simulink model "ECU_B_Enumerated_Error_Code_Generator"  (R2022a)
settings: Solver=VariableStepAuto  StartTime=0.0  StopTime=10  RelTol=1e-3
(part 1 of 2)
settings Model: Creator=maxju  LastModifiedBy=maxju

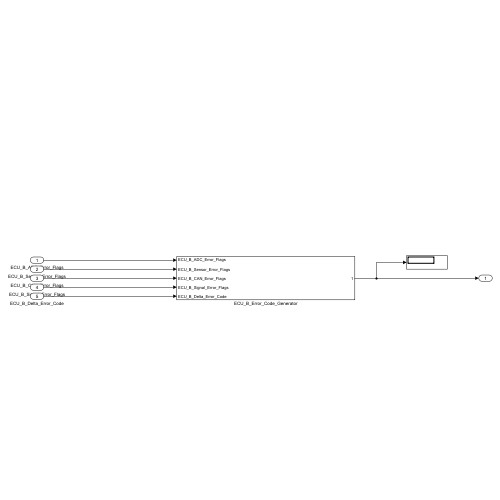
[thumbnail: Simulink's stored preview of the top-level diagram]
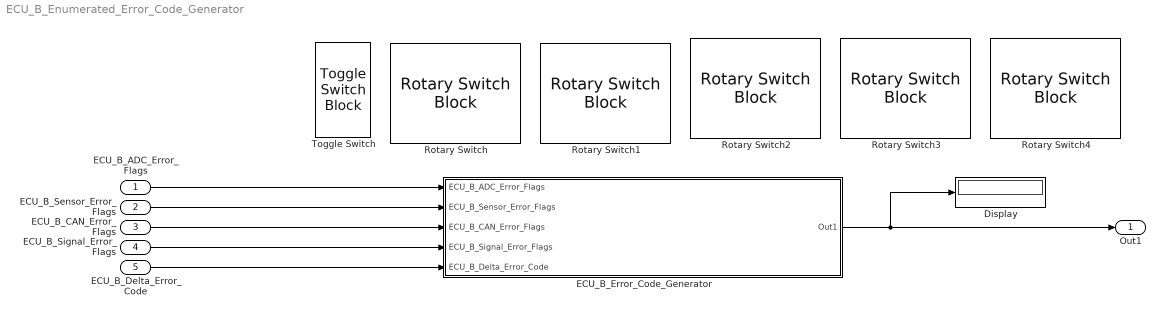
== system ECU_B_Enumerated_Error_Code_Generator ==
  ECU_B_ADC_Error_Flags : Inport
  ECU_B_Sensor_Error_Flags : Inport  Port=2
  ECU_B_CAN_Error_Flags : Inport  Port=3
  ECU_B_Signal_Error_Flags : Inport  Port=4
  ECU_B_Delta_Error_Code : Inport  Port=5
  Display : Display
  ECU_B_Error_Code_Generator : Subsystem
  Rotary Switch{,1..4} (5 alike) : RotarySwitchBlock
  Toggle Switch : ToggleSwitchBlock
      settings: Values={{'Off', 'On'}, [0 1]}
  Out1 : Outport
  wires:
  ECU_B_Signal_Error_Flags/1 -> ECU_B_Error_Code_Generator/4(ECU_B_Signal_Error_Flags)
  ECU_B_CAN_Error_Flags/1 -> ECU_B_Error_Code_Generator/3(ECU_B_CAN_Error_Flags)
  ECU_B_Sensor_Error_Flags/1 -> ECU_B_Error_Code_Generator/2(ECU_B_Sensor_Error_Flags)
  ECU_B_Error_Code_Generator/1(Out1) -> Out1/1, Display/1
  ECU_B_Delta_Error_Code/1 -> ECU_B_Error_Code_Generator/5(ECU_B_Delta_Error_Code)
  ECU_B_ADC_Error_Flags/1 -> ECU_B_Error_Code_Generator/1(ECU_B_ADC_Error_Flags)

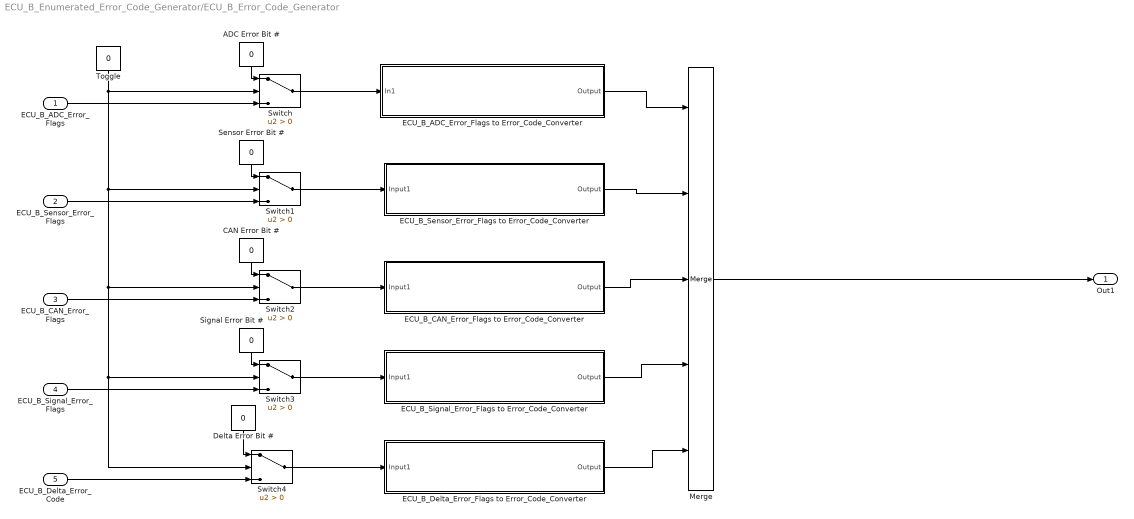
== system ECU_B_Enumerated_Error_Code_Generator/ECU_B_Error_Code_Generator ==
  ECU_B_ADC_Error_Flags : Inport
  ECU_B_Sensor_Error_Flags : Inport  Port=2
  ECU_B_CAN_Error_Flags : Inport  Port=3
  ECU_B_Signal_Error_Flags : Inport  Port=4
  ECU_B_Delta_Error_Code : Inport  Port=5
  ADC Error Bit # : Constant  Value=0
  CAN Error Bit # : Constant  Value=0
  Delta Error Bit # : Constant  Value=0
  ECU_B_ADC_Error_Flags to Error_Code_Converter : Subsystem
  ECU_B_CAN_Error_Flags to Error_Code_Converter : Subsystem
  ECU_B_Delta_Error_Flags to Error_Code_Converter : Subsystem
  ECU_B_Sensor_Error_Flags to Error_Code_Converter : Subsystem
  ECU_B_Signal_Error_Flags to Error_Code_Converter : Subsystem
  Merge : Merge  Inputs=5
  Sensor Error Bit # : Constant  Value=0
  Signal Error Bit # : Constant  Value=0
  Switch{,1..4} (5 alike) : Switch  Criteria=u2 > Threshold  SaturateOnIntegerOverflow=off  InputSameDT=off
  Toggle : Constant  Value=0
  Out1 : Outport
  wires:
  Merge/1 -> Out1/1
  ECU_B_ADC_Error_Flags to Error_Code_Converter/1(Output) -> Merge/1
  CAN Error Bit #/1 -> Switch2/1
  Switch1/1 -> ECU_B_Sensor_Error_Flags to Error_Code_Converter/1(Input1)
  Toggle/1 -> Switch2/2, Switch3/2, Switch4/2, Switch1/2, Switch/2
  ECU_B_Sensor_Error_Flags to Error_Code_Converter/1(Output) -> Merge/2
  ECU_B_CAN_Error_Flags to Error_Code_Converter/1(Output) -> Merge/3
  Switch/1 -> ECU_B_ADC_Error_Flags to Error_Code_Converter/1(In1)
  ECU_B_Signal_Error_Flags to Error_Code_Converter/1(Output) -> Merge/4
  Delta Error Bit #/1 -> Switch4/1
  ADC Error Bit #/1 -> Switch/1
  ECU_B_Delta_Error_Flags to Error_Code_Converter/1(Output) -> Merge/5
  ECU_B_Sensor_Error_Flags/1 -> Switch1/3
  ECU_B_ADC_Error_Flags/1 -> Switch/3
  Sensor Error Bit #/1 -> Switch1/1
  Signal Error Bit #/1 -> Switch3/1
  Switch2/1 -> ECU_B_CAN_Error_Flags to Error_Code_Converter/1(Input1)
  Switch3/1 -> ECU_B_Signal_Error_Flags to Error_Code_Converter/1(Input1)
  Switch4/1 -> ECU_B_Delta_Error_Flags to Error_Code_Converter/1(Input1)
  ECU_B_Signal_Error_Flags/1 -> Switch3/3
  ECU_B_CAN_Error_Flags/1 -> Switch2/3
  ECU_B_Delta_Error_Code/1 -> Switch4/3

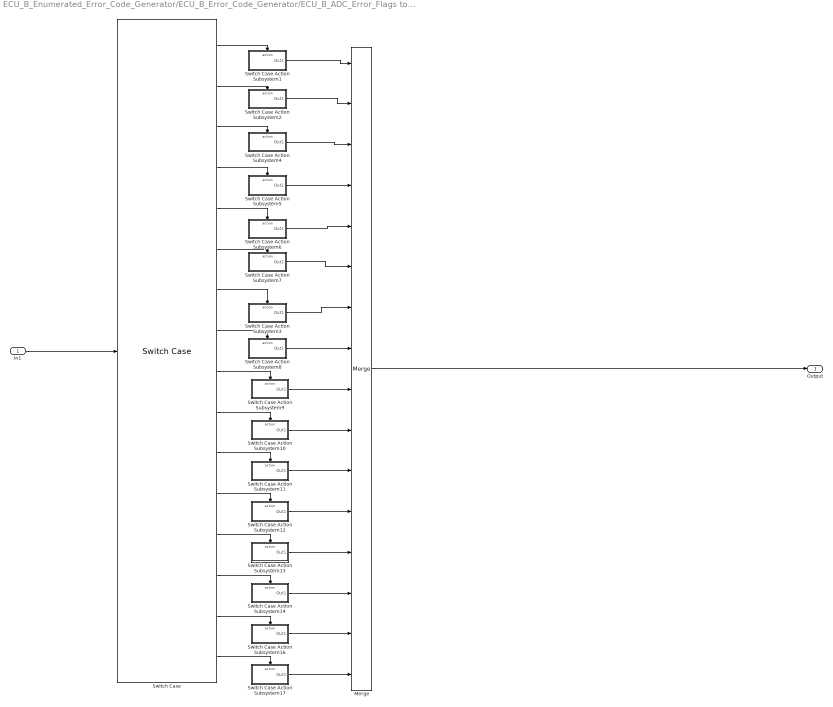
== system ECU_B_Enumerated_Error_Code_Generator/ECU_B_Error_Code_Generator/ECU_B_ADC_Error_Flags to Error_Code_Converter ==
  In1 : Inport
  Merge : Merge  Inputs=16
  Switch Case : SwitchCase  CaseConditions={1,2,3,4,5,6,7,8,9,10,11,12,13,14,15,16}  ShowDefaultCase=off
  Switch Case Action Subsystem1 : Subsystem  TreatAsAtomicUnit=on
  Switch Case Action Subsystem10 : Subsystem  TreatAsAtomicUnit=on
  Switch Case Action Subsystem11 : Subsystem  TreatAsAtomicUnit=on
  Switch Case Action Subsystem12 : Subsystem  TreatAsAtomicUnit=on
  Switch Case Action Subsystem13 : Subsystem  TreatAsAtomicUnit=on
  Switch Case Action Subsystem14 : Subsystem  TreatAsAtomicUnit=on
  Switch Case Action Subsystem16 : Subsystem  TreatAsAtomicUnit=on
  Switch Case Action Subsystem17 : Subsystem  TreatAsAtomicUnit=on
  Switch Case Action Subsystem2 : Subsystem  TreatAsAtomicUnit=on
  Switch Case Action Subsystem3 : Subsystem  TreatAsAtomicUnit=on
  Switch Case Action Subsystem4 : Subsystem  TreatAsAtomicUnit=on
  Switch Case Action Subsystem5 : Subsystem  TreatAsAtomicUnit=on
  Switch Case Action Subsystem6 : Subsystem  TreatAsAtomicUnit=on
  Switch Case Action Subsystem7 : Subsystem  TreatAsAtomicUnit=on
  Switch Case Action Subsystem8 : Subsystem  TreatAsAtomicUnit=on
  Switch Case Action Subsystem9 : Subsystem  TreatAsAtomicUnit=on
  Output : Outport
  wires:
  Switch Case/1 -> Switch Case Action Subsystem1/Action
  Switch Case/11 -> Switch Case Action Subsystem11/Action
  Switch Case/15 -> Switch Case Action Subsystem16/Action
  Switch Case Action Subsystem12/1(Out1) -> Merge/12
  Switch Case Action Subsystem17/1(Out1) -> Merge/16
  Switch Case/8 -> Switch Case Action Subsystem8/Action
  Switch Case Action Subsystem3/1(Out1) -> Merge/7
  Switch Case Action Subsystem14/1(Out1) -> Merge/14
  Switch Case/2 -> Switch Case Action Subsystem2/Action
  Switch Case/6 -> Switch Case Action Subsystem7/Action
  Switch Case Action Subsystem8/1(Out1) -> Merge/8
  Switch Case Action Subsystem10/1(Out1) -> Merge/10
  Switch Case Action Subsystem1/1(Out1) -> Merge/1
  Switch Case/9 -> Switch Case Action Subsystem9/Action
  Switch Case Action Subsystem5/1(Out1) -> Merge/4
  Switch Case Action Subsystem13/1(Out1) -> Merge/13
  Switch Case Action Subsystem11/1(Out1) -> Merge/11
  Switch Case/16 -> Switch Case Action Subsystem17/Action
  In1/1 -> Switch Case/1
  Switch Case/3 -> Switch Case Action Subsystem4/Action
  Switch Case/4 -> Switch Case Action Subsystem5/Action
  Switch Case/14 -> Switch Case Action Subsystem14/Action
  Switch Case Action Subsystem6/1(Out1) -> Merge/5
  Switch Case/5 -> Switch Case Action Subsystem6/Action
  Switch Case Action Subsystem2/1(Out1) -> Merge/2
  Switch Case/12 -> Switch Case Action Subsystem12/Action
  Switch Case Action Subsystem4/1(Out1) -> Merge/3
  Switch Case Action Subsystem9/1(Out1) -> Merge/9
  Switch Case/7 -> Switch Case Action Subsystem3/Action
  Switch Case/13 -> Switch Case Action Subsystem13/Action
  Switch Case Action Subsystem7/1(Out1) -> Merge/6
  Switch Case/10 -> Switch Case Action Subsystem10/Action
  Switch Case Action Subsystem16/1(Out1) -> Merge/15
  Merge/1 -> Output/1

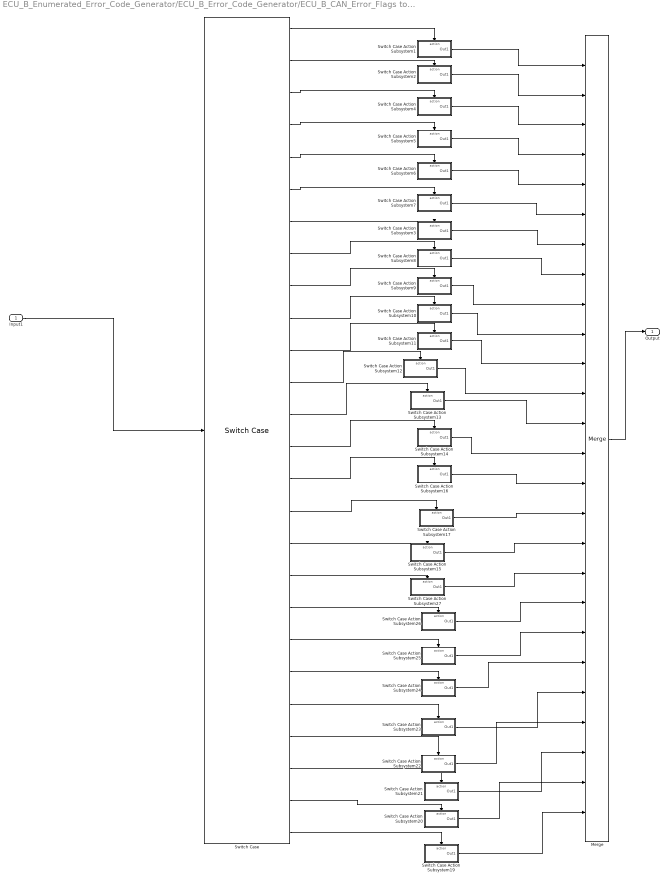
== system ECU_B_Enumerated_Error_Code_Generator/ECU_B_Error_Code_Generator/ECU_B_CAN_Error_Flags to Error_Code_Converter ==
  Input1 : Inport
  Merge : Merge  Inputs=26
  Switch Case : SwitchCase  CaseConditions={1,2,3,4,5,6,7,8,9,10,11,12,13,14,15,16,17,18,19,20,21,22,23,24,25,26}  ShowDefaultCase=off
  Switch Case Action Subsystem1 : Subsystem  TreatAsAtomicUnit=on
  Switch Case Action Subsystem10 : Subsystem  TreatAsAtomicUnit=on
  Switch Case Action Subsystem11 : Subsystem  TreatAsAtomicUnit=on
  Switch Case Action Subsystem12 : Subsystem  TreatAsAtomicUnit=on
  Switch Case Action Subsystem13 : Subsystem  TreatAsAtomicUnit=on
  Switch Case Action Subsystem14 : Subsystem  TreatAsAtomicUnit=on
  Switch Case Action Subsystem15 : Subsystem  TreatAsAtomicUnit=on
  Switch Case Action Subsystem16 : Subsystem  TreatAsAtomicUnit=on
  Switch Case Action Subsystem17 : Subsystem  TreatAsAtomicUnit=on
  Switch Case Action Subsystem19 : Subsystem  TreatAsAtomicUnit=on
  Switch Case Action Subsystem2 : Subsystem  TreatAsAtomicUnit=on
  Switch Case Action Subsystem20 : Subsystem  TreatAsAtomicUnit=on
  Switch Case Action Subsystem21 : Subsystem  TreatAsAtomicUnit=on
  Switch Case Action Subsystem22 : Subsystem  TreatAsAtomicUnit=on
  Switch Case Action Subsystem23 : Subsystem  TreatAsAtomicUnit=on
  Switch Case Action Subsystem24 : Subsystem  TreatAsAtomicUnit=on
  Switch Case Action Subsystem25 : Subsystem  TreatAsAtomicUnit=on
  Switch Case Action Subsystem26 : Subsystem  TreatAsAtomicUnit=on
  Switch Case Action Subsystem27 : Subsystem  TreatAsAtomicUnit=on
  Switch Case Action Subsystem3 : Subsystem  TreatAsAtomicUnit=on
  Switch Case Action Subsystem4 : Subsystem  TreatAsAtomicUnit=on
  Switch Case Action Subsystem5 : Subsystem  TreatAsAtomicUnit=on
  Switch Case Action Subsystem6 : Subsystem  TreatAsAtomicUnit=on
  Switch Case Action Subsystem7 : Subsystem  TreatAsAtomicUnit=on
  Switch Case Action Subsystem8 : Subsystem  TreatAsAtomicUnit=on
  Switch Case Action Subsystem9 : Subsystem  TreatAsAtomicUnit=on
  Output : Outport
  wires:
  Switch Case/1 -> Switch Case Action Subsystem1/Action
  Switch Case/11 -> Switch Case Action Subsystem11/Action
  Switch Case/15 -> Switch Case Action Subsystem16/Action
  Switch Case Action Subsystem12/1(Out1) -> Merge/12
  Switch Case Action Subsystem17/1(Out1) -> Merge/16
  Switch Case/8 -> Switch Case Action Subsystem8/Action
  Switch Case Action Subsystem3/1(Out1) -> Merge/7
  Switch Case Action Subsystem14/1(Out1) -> Merge/14
  Switch Case/2 -> Switch Case Action Subsystem2/Action
  Switch Case/6 -> Switch Case Action Subsystem7/Action
  Switch Case Action Subsystem8/1(Out1) -> Merge/8
  Switch Case Action Subsystem10/1(Out1) -> Merge/10
  Switch Case Action Subsystem1/1(Out1) -> Merge/1
  Switch Case/9 -> Switch Case Action Subsystem9/Action
  Switch Case Action Subsystem5/1(Out1) -> Merge/4
  Switch Case Action Subsystem13/1(Out1) -> Merge/13
  Switch Case Action Subsystem11/1(Out1) -> Merge/11
  Merge/1 -> Output/1
  Switch Case/16 -> Switch Case Action Subsystem17/Action
  Input1/1 -> Switch Case/1
  Switch Case/3 -> Switch Case Action Subsystem4/Action
  Switch Case/4 -> Switch Case Action Subsystem5/Action
  Switch Case/14 -> Switch Case Action Subsystem14/Action
  Switch Case Action Subsystem6/1(Out1) -> Merge/5
  Switch Case/5 -> Switch Case Action Subsystem6/Action
  Switch Case Action Subsystem2/1(Out1) -> Merge/2
  Switch Case/12 -> Switch Case Action Subsystem12/Action
  Switch Case Action Subsystem4/1(Out1) -> Merge/3
  Switch Case Action Subsystem9/1(Out1) -> Merge/9
  Switch Case/7 -> Switch Case Action Subsystem3/Action
  Switch Case/13 -> Switch Case Action Subsystem13/Action
  Switch Case Action Subsystem7/1(Out1) -> Merge/6
  Switch Case/10 -> Switch Case Action Subsystem10/Action
  Switch Case Action Subsystem16/1(Out1) -> Merge/15
  Switch Case/17 -> Switch Case Action Subsystem15/Action
  Switch Case Action Subsystem15/1(Out1) -> Merge/17
  Switch Case/18 -> Switch Case Action Subsystem27/Action
  Switch Case Action Subsystem27/1(Out1) -> Merge/18
  Switch Case/19 -> Switch Case Action Subsystem26/Action
  Switch Case Action Subsystem26/1(Out1) -> Merge/19
  Switch Case/20 -> Switch Case Action Subsystem25/Action
  Switch Case Action Subsystem25/1(Out1) -> Merge/20
  Switch Case/21 -> Switch Case Action Subsystem24/Action
  Switch Case Action Subsystem24/1(Out1) -> Merge/21
  Switch Case/22 -> Switch Case Action Subsystem23/Action
  Switch Case Action Subsystem23/1(Out1) -> Merge/22
  Switch Case/23 -> Switch Case Action Subsystem22/Action
  Switch Case Action Subsystem22/1(Out1) -> Merge/23
  Switch Case/24 -> Switch Case Action Subsystem21/Action
  Switch Case Action Subsystem21/1(Out1) -> Merge/24
  Switch Case/25 -> Switch Case Action Subsystem20/Action
  Switch Case Action Subsystem20/1(Out1) -> Merge/25
  Switch Case/26 -> Switch Case Action Subsystem19/Action
  Switch Case Action Subsystem19/1(Out1) -> Merge/26

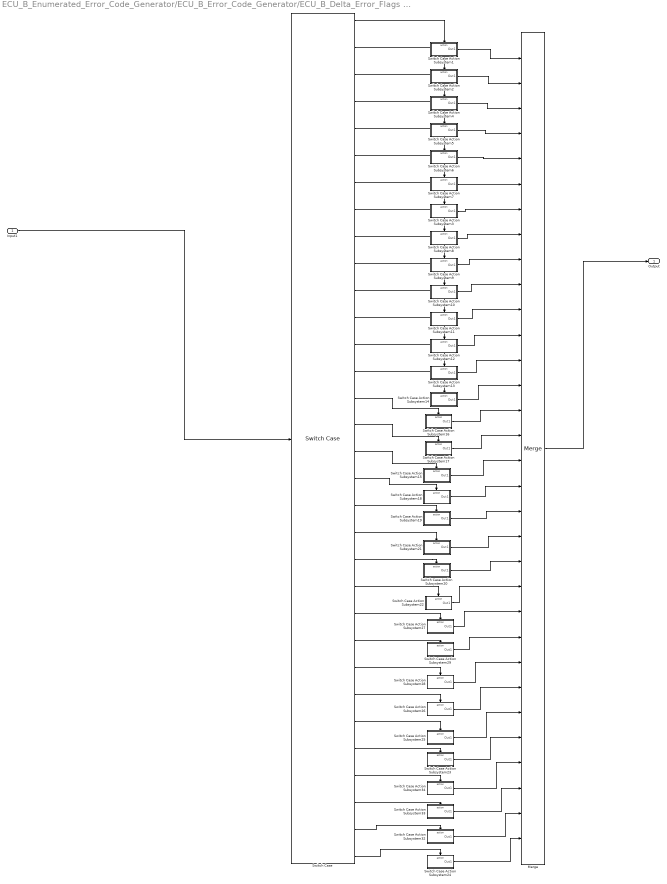
== system ECU_B_Enumerated_Error_Code_Generator/ECU_B_Error_Code_Generator/ECU_B_Delta_Error_Flags to Error_Code_Converter ==
  Input1 : Inport
  Merge : Merge  Inputs=32
  Switch Case : SwitchCase  CaseConditions={1,2,3,4,5,6,7,8,9,10,11,12,13,14,15,16,17,18,19,20,21,22,23,24,25,26,27,28,29,30,31,32}  ShowDefaultCase=off
  Switch Case Action Subsystem1 : Subsystem  TreatAsAtomicUnit=on
  Switch Case Action Subsystem10 : Subsystem  TreatAsAtomicUnit=on
  Switch Case Action Subsystem11 : Subsystem  TreatAsAtomicUnit=on
  Switch Case Action Subsystem12 : Subsystem  TreatAsAtomicUnit=on
  Switch Case Action Subsystem13 : Subsystem  TreatAsAtomicUnit=on
  Switch Case Action Subsystem14 : Subsystem  TreatAsAtomicUnit=on
  Switch Case Action Subsystem15 : Subsystem  TreatAsAtomicUnit=on
  Switch Case Action Subsystem16 : Subsystem  TreatAsAtomicUnit=on
  Switch Case Action Subsystem17 : Subsystem  TreatAsAtomicUnit=on
  Switch Case Action Subsystem18 : Subsystem  TreatAsAtomicUnit=on
  Switch Case Action Subsystem19 : Subsystem  TreatAsAtomicUnit=on
  Switch Case Action Subsystem2 : Subsystem  TreatAsAtomicUnit=on
  Switch Case Action Subsystem20 : Subsystem  TreatAsAtomicUnit=on
  Switch Case Action Subsystem21 : Subsystem  TreatAsAtomicUnit=on
  Switch Case Action Subsystem22 : Subsystem  TreatAsAtomicUnit=on
  Switch Case Action Subsystem23 : Subsystem  TreatAsAtomicUnit=on
  Switch Case Action Subsystem24 : Subsystem  TreatAsAtomicUnit=on
  Switch Case Action Subsystem25 : Subsystem  TreatAsAtomicUnit=on
  Switch Case Action Subsystem26 : Subsystem  TreatAsAtomicUnit=on
  Switch Case Action Subsystem27 : Subsystem  TreatAsAtomicUnit=on
  Switch Case Action Subsystem28 : Subsystem  TreatAsAtomicUnit=on
  Switch Case Action Subsystem29 : Subsystem  TreatAsAtomicUnit=on
  Switch Case Action Subsystem3 : Subsystem  TreatAsAtomicUnit=on
  Switch Case Action Subsystem32 : Subsystem  TreatAsAtomicUnit=on
  Switch Case Action Subsystem33 : Subsystem  TreatAsAtomicUnit=on
  Switch Case Action Subsystem34 : Subsystem  TreatAsAtomicUnit=on
  Switch Case Action Subsystem4 : Subsystem  TreatAsAtomicUnit=on
  Switch Case Action Subsystem5 : Subsystem  TreatAsAtomicUnit=on
  Switch Case Action Subsystem6 : Subsystem  TreatAsAtomicUnit=on
  Switch Case Action Subsystem7 : Subsystem  TreatAsAtomicUnit=on
  Switch Case Action Subsystem8 : Subsystem  TreatAsAtomicUnit=on
  Switch Case Action Subsystem9 : Subsystem  TreatAsAtomicUnit=on
  Output : Outport
  wires:
  Switch Case/1 -> Switch Case Action Subsystem1/Action
  Switch Case/11 -> Switch Case Action Subsystem11/Action
  Switch Case/15 -> Switch Case Action Subsystem16/Action
  Switch Case Action Subsystem12/1(Out1) -> Merge/12
  Switch Case Action Subsystem17/1(Out1) -> Merge/16
  Switch Case/8 -> Switch Case Action Subsystem8/Action
  Switch Case Action Subsystem3/1(Out1) -> Merge/7
  Switch Case Action Subsystem14/1(Out1) -> Merge/14
  Switch Case/2 -> Switch Case Action Subsystem2/Action
  Switch Case/6 -> Switch Case Action Subsystem7/Action
  Switch Case Action Subsystem8/1(Out1) -> Merge/8
  Switch Case Action Subsystem10/1(Out1) -> Merge/10
  Switch Case Action Subsystem1/1(Out1) -> Merge/1
  Switch Case/9 -> Switch Case Action Subsystem9/Action
  Switch Case Action Subsystem5/1(Out1) -> Merge/4
  Switch Case Action Subsystem13/1(Out1) -> Merge/13
  Switch Case Action Subsystem11/1(Out1) -> Merge/11
  Merge/1 -> Output/1
  Switch Case/16 -> Switch Case Action Subsystem17/Action
  Input1/1 -> Switch Case/1
  Switch Case/3 -> Switch Case Action Subsystem4/Action
  Switch Case/4 -> Switch Case Action Subsystem5/Action
  Switch Case/14 -> Switch Case Action Subsystem14/Action
  Switch Case Action Subsystem6/1(Out1) -> Merge/5
  Switch Case/5 -> Switch Case Action Subsystem6/Action
  Switch Case Action Subsystem2/1(Out1) -> Merge/2
  Switch Case/12 -> Switch Case Action Subsystem12/Action
  Switch Case Action Subsystem4/1(Out1) -> Merge/3
  Switch Case Action Subsystem9/1(Out1) -> Merge/9
  Switch Case/7 -> Switch Case Action Subsystem3/Action
  Switch Case/13 -> Switch Case Action Subsystem13/Action
  Switch Case Action Subsystem7/1(Out1) -> Merge/6
  Switch Case/10 -> Switch Case Action Subsystem10/Action
  Switch Case Action Subsystem16/1(Out1) -> Merge/15
  Switch Case/17 -> Switch Case Action Subsystem15/Action
  Switch Case Action Subsystem15/1(Out1) -> Merge/17
  Switch Case/18 -> Switch Case Action Subsystem18/Action
  Switch Case Action Subsystem18/1(Out1) -> Merge/18
  Switch Case/19 -> Switch Case Action Subsystem19/Action
  Switch Case Action Subsystem19/1(Out1) -> Merge/19
  Switch Case/20 -> Switch Case Action Subsystem21/Action
  Switch Case Action Subsystem21/1(Out1) -> Merge/20
  Switch Case/21 -> Switch Case Action Subsystem20/Action
  Switch Case Action Subsystem20/1(Out1) -> Merge/21
  Switch Case/22 -> Switch Case Action Subsystem22/Action
  Switch Case Action Subsystem22/1(Out1) -> Merge/22
  Switch Case/23 -> Switch Case Action Subsystem27/Action
  Switch Case Action Subsystem27/1(Out1) -> Merge/23
  Switch Case/24 -> Switch Case Action Subsystem29/Action
  Switch Case Action Subsystem29/1(Out1) -> Merge/24
  Switch Case/25 -> Switch Case Action Subsystem28/Action
  Switch Case Action Subsystem28/1(Out1) -> Merge/25
  Switch Case/26 -> Switch Case Action Subsystem26/Action
  Switch Case Action Subsystem26/1(Out1) -> Merge/26
  Switch Case/27 -> Switch Case Action Subsystem25/Action
  Switch Case Action Subsystem25/1(Out1) -> Merge/27
  Switch Case/28 -> Switch Case Action Subsystem23/Action
  Switch Case Action Subsystem23/1(Out1) -> Merge/28
  Switch Case/29 -> Switch Case Action Subsystem34/Action
  Switch Case Action Subsystem34/1(Out1) -> Merge/29
  Switch Case/30 -> Switch Case Action Subsystem33/Action
  Switch Case Action Subsystem33/1(Out1) -> Merge/30
  Switch Case/31 -> Switch Case Action Subsystem32/Action
  Switch Case Action Subsystem32/1(Out1) -> Merge/31
  Switch Case/32 -> Switch Case Action Subsystem24/Action
  Switch Case Action Subsystem24/1(Out1) -> Merge/32

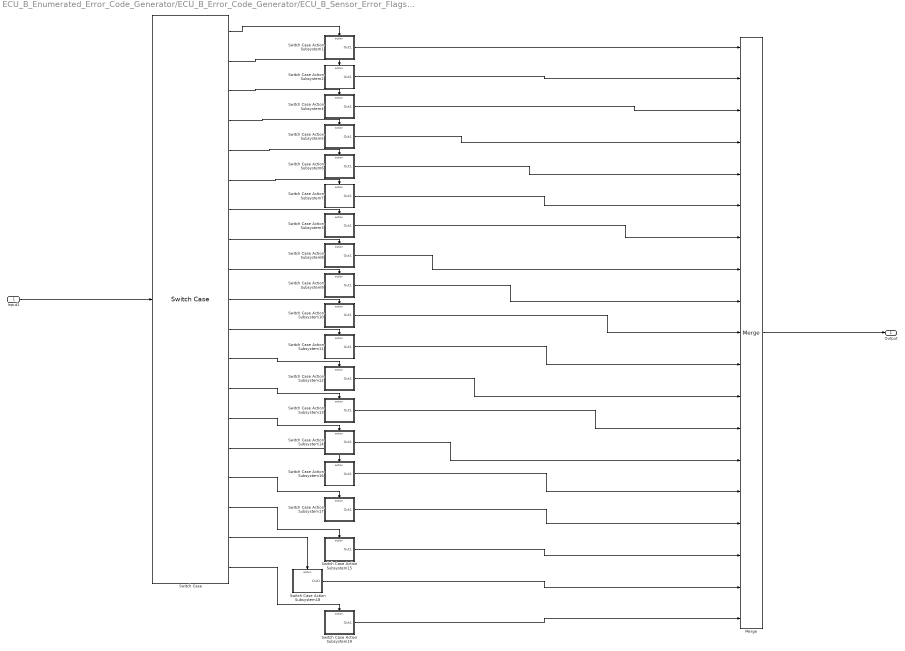
== system ECU_B_Enumerated_Error_Code_Generator/ECU_B_Error_Code_Generator/ECU_B_Sensor_Error_Flags to Error_Code_Converter ==
  Input1 : Inport
  Merge : Merge  Inputs=19
  Switch Case : SwitchCase  CaseConditions={1,2,3,4,5,6,7,8,9,10,11,12,13,14,15,16,17,18,19}  ShowDefaultCase=off
  Switch Case Action Subsystem1 : Subsystem  TreatAsAtomicUnit=on
  Switch Case Action Subsystem10 : Subsystem  TreatAsAtomicUnit=on
  Switch Case Action Subsystem11 : Subsystem  TreatAsAtomicUnit=on
  Switch Case Action Subsystem12 : Subsystem  TreatAsAtomicUnit=on
  Switch Case Action Subsystem13 : Subsystem  TreatAsAtomicUnit=on
  Switch Case Action Subsystem14 : Subsystem  TreatAsAtomicUnit=on
  Switch Case Action Subsystem15 : Subsystem  TreatAsAtomicUnit=on
  Switch Case Action Subsystem16 : Subsystem  TreatAsAtomicUnit=on
  Switch Case Action Subsystem17 : Subsystem  TreatAsAtomicUnit=on
  Switch Case Action Subsystem18 : Subsystem  TreatAsAtomicUnit=on
  Switch Case Action Subsystem19 : Subsystem  TreatAsAtomicUnit=on
  Switch Case Action Subsystem2 : Subsystem  TreatAsAtomicUnit=on
  Switch Case Action Subsystem3 : Subsystem  TreatAsAtomicUnit=on
  Switch Case Action Subsystem4 : Subsystem  TreatAsAtomicUnit=on
  Switch Case Action Subsystem5 : Subsystem  TreatAsAtomicUnit=on
  Switch Case Action Subsystem6 : Subsystem  TreatAsAtomicUnit=on
  Switch Case Action Subsystem7 : Subsystem  TreatAsAtomicUnit=on
  Switch Case Action Subsystem8 : Subsystem  TreatAsAtomicUnit=on
  Switch Case Action Subsystem9 : Subsystem  TreatAsAtomicUnit=on
  Output : Outport
  wires:
  Switch Case Action Subsystem5/1(Out1) -> Merge/4
  Switch Case Action Subsystem1/1(Out1) -> Merge/1
  Switch Case Action Subsystem17/1(Out1) -> Merge/16
  Switch Case Action Subsystem3/1(Out1) -> Merge/7
  Switch Case Action Subsystem10/1(Out1) -> Merge/10
  Switch Case Action Subsystem14/1(Out1) -> Merge/14
  Switch Case/2 -> Switch Case Action Subsystem2/Action
  Switch Case/1 -> Switch Case Action Subsystem1/Action
  Switch Case Action Subsystem13/1(Out1) -> Merge/13
  Switch Case Action Subsystem11/1(Out1) -> Merge/11
  Merge/1 -> Output/1
  Switch Case/15 -> Switch Case Action Subsystem16/Action
  Switch Case/16 -> Switch Case Action Subsystem17/Action
  Input1/1 -> Switch Case/1
  Switch Case/3 -> Switch Case Action Subsystem4/Action
  Switch Case/4 -> Switch Case Action Subsystem5/Action
  Switch Case Action Subsystem6/1(Out1) -> Merge/5
  Switch Case/6 -> Switch Case Action Subsystem7/Action
  Switch Case/5 -> Switch Case Action Subsystem6/Action
  Switch Case Action Subsystem2/1(Out1) -> Merge/2
  Switch Case/11 -> Switch Case Action Subsystem11/Action
  Switch Case/12 -> Switch Case Action Subsystem12/Action
  Switch Case Action Subsystem4/1(Out1) -> Merge/3
  Switch Case Action Subsystem9/1(Out1) -> Merge/9
  Switch Case/8 -> Switch Case Action Subsystem8/Action
  Switch Case/7 -> Switch Case Action Subsystem3/Action
  Switch Case/14 -> Switch Case Action Subsystem14/Action
  Switch Case/13 -> Switch Case Action Subsystem13/Action
  Switch Case Action Subsystem7/1(Out1) -> Merge/6
  Switch Case/17 -> Switch Case Action Subsystem15/Action
  Switch Case/19 -> Switch Case Action Subsystem19/Action
  Switch Case Action Subsystem18/1(Out1) -> Merge/18
  Switch Case Action Subsystem15/1(Out1) -> Merge/17
  Switch Case/9 -> Switch Case Action Subsystem9/Action
  Switch Case/10 -> Switch Case Action Subsystem10/Action
  Switch Case Action Subsystem12/1(Out1) -> Merge/12
  Switch Case Action Subsystem19/1(Out1) -> Merge/19
  Switch Case Action Subsystem8/1(Out1) -> Merge/8
  Switch Case/18 -> Switch Case Action Subsystem18/Action
  Switch Case Action Subsystem16/1(Out1) -> Merge/15

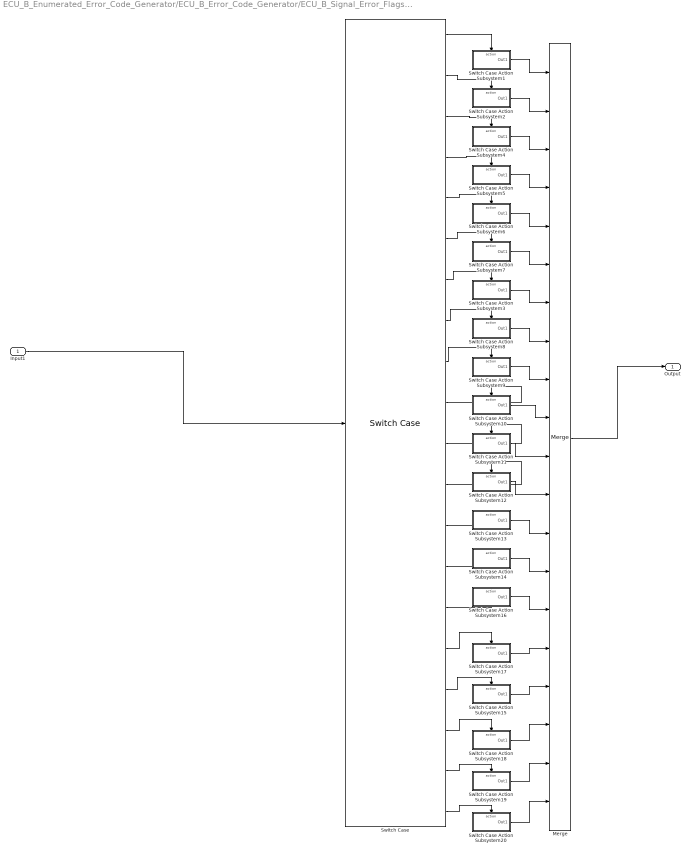
== system ECU_B_Enumerated_Error_Code_Generator/ECU_B_Error_Code_Generator/ECU_B_Signal_Error_Flags to Error_Code_Converter ==
  Input1 : Inport
  Merge : Merge  Inputs=20
  Switch Case : SwitchCase  CaseConditions={1,2,3,4,5,6,7,8,9,10,11,12,13,14,15,16,17,18,19,20}  ShowDefaultCase=off
  Switch Case Action Subsystem1 : Subsystem  TreatAsAtomicUnit=on
  Switch Case Action Subsystem10 : Subsystem  TreatAsAtomicUnit=on
  Switch Case Action Subsystem11 : Subsystem  TreatAsAtomicUnit=on
  Switch Case Action Subsystem12 : Subsystem  TreatAsAtomicUnit=on
  Switch Case Action Subsystem13 : Subsystem  TreatAsAtomicUnit=on
  Switch Case Action Subsystem14 : Subsystem  TreatAsAtomicUnit=on
  Switch Case Action Subsystem15 : Subsystem  TreatAsAtomicUnit=on
  Switch Case Action Subsystem16 : Subsystem  TreatAsAtomicUnit=on
  Switch Case Action Subsystem17 : Subsystem  TreatAsAtomicUnit=on
  Switch Case Action Subsystem18 : Subsystem  TreatAsAtomicUnit=on
  Switch Case Action Subsystem19 : Subsystem  TreatAsAtomicUnit=on
  Switch Case Action Subsystem2 : Subsystem  TreatAsAtomicUnit=on
  Switch Case Action Subsystem20 : Subsystem  TreatAsAtomicUnit=on
  Switch Case Action Subsystem3 : Subsystem  TreatAsAtomicUnit=on
  Switch Case Action Subsystem4 : Subsystem  TreatAsAtomicUnit=on
  Switch Case Action Subsystem5 : Subsystem  TreatAsAtomicUnit=on
  Switch Case Action Subsystem6 : Subsystem  TreatAsAtomicUnit=on
  Switch Case Action Subsystem7 : Subsystem  TreatAsAtomicUnit=on
  Switch Case Action Subsystem8 : Subsystem  TreatAsAtomicUnit=on
  Switch Case Action Subsystem9 : Subsystem  TreatAsAtomicUnit=on
  Output : Outport
  wires:
  Switch Case/1 -> Switch Case Action Subsystem1/Action
  Switch Case/11 -> Switch Case Action Subsystem11/Action
  Switch Case/15 -> Switch Case Action Subsystem16/Action
  Switch Case Action Subsystem12/1(Out1) -> Merge/12
  Switch Case Action Subsystem17/1(Out1) -> Merge/16
  Switch Case/8 -> Switch Case Action Subsystem8/Action
  Switch Case Action Subsystem3/1(Out1) -> Merge/7
  Switch Case Action Subsystem14/1(Out1) -> Merge/14
  Switch Case/2 -> Switch Case Action Subsystem2/Action
  Switch Case/6 -> Switch Case Action Subsystem7/Action
  Switch Case Action Subsystem8/1(Out1) -> Merge/8
  Switch Case Action Subsystem10/1(Out1) -> Merge/10
  Switch Case Action Subsystem1/1(Out1) -> Merge/1
  Switch Case/9 -> Switch Case Action Subsystem9/Action
  Switch Case Action Subsystem5/1(Out1) -> Merge/4
  Switch Case Action Subsystem13/1(Out1) -> Merge/13
  Switch Case Action Subsystem11/1(Out1) -> Merge/11
  Merge/1 -> Output/1
  Switch Case/16 -> Switch Case Action Subsystem17/Action
  Input1/1 -> Switch Case/1
  Switch Case/3 -> Switch Case Action Subsystem4/Action
  Switch Case/4 -> Switch Case Action Subsystem5/Action
  Switch Case/14 -> Switch Case Action Subsystem14/Action
  Switch Case Action Subsystem6/1(Out1) -> Merge/5
  Switch Case/5 -> Switch Case Action Subsystem6/Action
  Switch Case Action Subsystem2/1(Out1) -> Merge/2
  Switch Case/12 -> Switch Case Action Subsystem12/Action
  Switch Case Action Subsystem4/1(Out1) -> Merge/3
  Switch Case Action Subsystem9/1(Out1) -> Merge/9
  Switch Case/7 -> Switch Case Action Subsystem3/Action
  Switch Case/13 -> Switch Case Action Subsystem13/Action
  Switch Case Action Subsystem7/1(Out1) -> Merge/6
  Switch Case/10 -> Switch Case Action Subsystem10/Action
  Switch Case Action Subsystem16/1(Out1) -> Merge/15
  Switch Case/17 -> Switch Case Action Subsystem15/Action
  Switch Case/18 -> Switch Case Action Subsystem18/Action
  Switch Case/19 -> Switch Case Action Subsystem19/Action
  Switch Case/20 -> Switch Case Action Subsystem20/Action
  Switch Case Action Subsystem15/1(Out1) -> Merge/17
  Switch Case Action Subsystem18/1(Out1) -> Merge/18
  Switch Case Action Subsystem19/1(Out1) -> Merge/19
  Switch Case Action Subsystem20/1(Out1) -> Merge/20

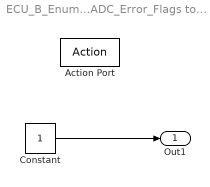
== system ECU_B_Enumerated_Error_Code_Generator/ECU_B_Error_Code_Generator/ECU_B_ADC_Error_Flags to Error_Code_Converter/Switch Case Action Subsystem1 ==
  Action Port : ActionPort  ActionPortLabel=case [ 1 ]:
  Constant : Constant
  Out1 : Outport  VectorParamsAs1DForOutWhenUnconnected=off
  wires:
  Constant/1 -> Out1/1

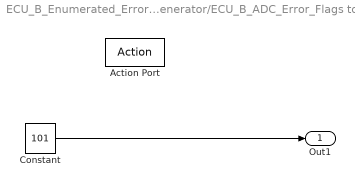
== system ECU_B_Enumerated_Error_Code_Generator/ECU_B_Error_Code_Generator/ECU_B_ADC_Error_Flags to Error_Code_Converter/Switch Case Action Subsystem10 ==
  Action Port : ActionPort  ActionPortLabel=case [ 10 ]:
  Constant : Constant  Value=101
  Out1 : Outport  VectorParamsAs1DForOutWhenUnconnected=off
  wires:
  Constant/1 -> Out1/1

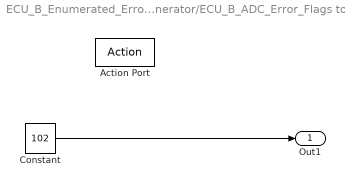
== system ECU_B_Enumerated_Error_Code_Generator/ECU_B_Error_Code_Generator/ECU_B_ADC_Error_Flags to Error_Code_Converter/Switch Case Action Subsystem11 ==
  Action Port : ActionPort  ActionPortLabel=case [ 11 ]:
  Constant : Constant  Value=102
  Out1 : Outport  VectorParamsAs1DForOutWhenUnconnected=off
  wires:
  Constant/1 -> Out1/1

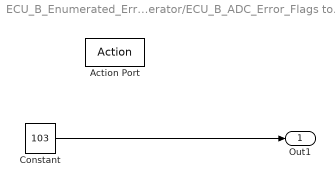
== system ECU_B_Enumerated_Error_Code_Generator/ECU_B_Error_Code_Generator/ECU_B_ADC_Error_Flags to Error_Code_Converter/Switch Case Action Subsystem12 ==
  Action Port : ActionPort  ActionPortLabel=case [ 12 ]:
  Constant : Constant  Value=103
  Out1 : Outport  VectorParamsAs1DForOutWhenUnconnected=off
  wires:
  Constant/1 -> Out1/1

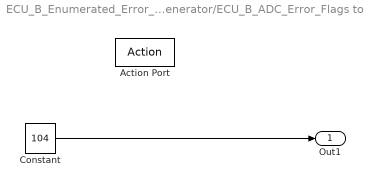
== system ECU_B_Enumerated_Error_Code_Generator/ECU_B_Error_Code_Generator/ECU_B_ADC_Error_Flags to Error_Code_Converter/Switch Case Action Subsystem13 ==
  Action Port : ActionPort  ActionPortLabel=case [ 13 ]:
  Constant : Constant  Value=104
  Out1 : Outport  VectorParamsAs1DForOutWhenUnconnected=off
  wires:
  Constant/1 -> Out1/1

== system ECU_B_Enumerated_Error_Code_Generator/ECU_B_Error_Code_Generator/ECU_B_ADC_Error_Flags to Error_Code_Converter/Switch Case Action Subsystem14 ==
  Action Port : ActionPort  ActionPortLabel=case [ 14 ]:
  Constant : Constant  Value=105
  Out1 : Outport  VectorParamsAs1DForOutWhenUnconnected=off
  wires:
  Constant/1 -> Out1/1

== system ECU_B_Enumerated_Error_Code_Generator/ECU_B_Error_Code_Generator/ECU_B_ADC_Error_Flags to Error_Code_Converter/Switch Case Action Subsystem16 ==
  Action Port : ActionPort  ActionPortLabel=case [ 15 ]:
  Constant : Constant  Value=106
  Out1 : Outport  VectorParamsAs1DForOutWhenUnconnected=off
  wires:
  Constant/1 -> Out1/1

== system ECU_B_Enumerated_Error_Code_Generator/ECU_B_Error_Code_Generator/ECU_B_ADC_Error_Flags to Error_Code_Converter/Switch Case Action Subsystem17 ==
  Action Port : ActionPort  ActionPortLabel=case [ 16 ]:
  Constant : Constant  Value=107
  Out1 : Outport  VectorParamsAs1DForOutWhenUnconnected=off
  wires:
  Constant/1 -> Out1/1

== system ECU_B_Enumerated_Error_Code_Generator/ECU_B_Error_Code_Generator/ECU_B_ADC_Error_Flags to Error_Code_Converter/Switch Case Action Subsystem2 ==
  Action Port : ActionPort  ActionPortLabel=case [ 2 ]:
  Constant : Constant  Value=2
  Out1 : Outport  VectorParamsAs1DForOutWhenUnconnected=off
  wires:
  Constant/1 -> Out1/1

== system ECU_B_Enumerated_Error_Code_Generator/ECU_B_Error_Code_Generator/ECU_B_ADC_Error_Flags to Error_Code_Converter/Switch Case Action Subsystem3 ==
  Action Port : ActionPort  ActionPortLabel=case [ 7 ]:
  Constant : Constant  Value=7
  Out1 : Outport  VectorParamsAs1DForOutWhenUnconnected=off
  wires:
  Constant/1 -> Out1/1

== system ECU_B_Enumerated_Error_Code_Generator/ECU_B_Error_Code_Generator/ECU_B_ADC_Error_Flags to Error_Code_Converter/Switch Case Action Subsystem4 ==
  Action Port : ActionPort  ActionPortLabel=case [ 3 ]:
  Constant : Constant  Value=3
  Out1 : Outport  VectorParamsAs1DForOutWhenUnconnected=off
  wires:
  Constant/1 -> Out1/1

== system ECU_B_Enumerated_Error_Code_Generator/ECU_B_Error_Code_Generator/ECU_B_ADC_Error_Flags to Error_Code_Converter/Switch Case Action Subsystem5 ==
  Action Port : ActionPort  ActionPortLabel=case [ 4 ]:
  Constant : Constant  Value=4
  Out1 : Outport  VectorParamsAs1DForOutWhenUnconnected=off
  wires:
  Constant/1 -> Out1/1

== system ECU_B_Enumerated_Error_Code_Generator/ECU_B_Error_Code_Generator/ECU_B_ADC_Error_Flags to Error_Code_Converter/Switch Case Action Subsystem6 ==
  Action Port : ActionPort  ActionPortLabel=case [ 5 ]:
  Constant : Constant  Value=5
  Out1 : Outport  VectorParamsAs1DForOutWhenUnconnected=off
  wires:
  Constant/1 -> Out1/1

== system ECU_B_Enumerated_Error_Code_Generator/ECU_B_Error_Code_Generator/ECU_B_ADC_Error_Flags to Error_Code_Converter/Switch Case Action Subsystem7 ==
  Action Port : ActionPort  ActionPortLabel=case [ 6 ]:
  Constant : Constant  Value=6
  Out1 : Outport  VectorParamsAs1DForOutWhenUnconnected=off
  wires:
  Constant/1 -> Out1/1

== system ECU_B_Enumerated_Error_Code_Generator/ECU_B_Error_Code_Generator/ECU_B_ADC_Error_Flags to Error_Code_Converter/Switch Case Action Subsystem8 ==
  Action Port : ActionPort  ActionPortLabel=case [ 8 ]:
  Constant : Constant  Value=8
  Out1 : Outport  VectorParamsAs1DForOutWhenUnconnected=off
  wires:
  Constant/1 -> Out1/1

== system ECU_B_Enumerated_Error_Code_Generator/ECU_B_Error_Code_Generator/ECU_B_ADC_Error_Flags to Error_Code_Converter/Switch Case Action Subsystem9 ==
  Action Port : ActionPort  ActionPortLabel=case [ 9 ]:
  Constant : Constant  Value=100
  Out1 : Outport  VectorParamsAs1DForOutWhenUnconnected=off
  wires:
  Constant/1 -> Out1/1

== system ECU_B_Enumerated_Error_Code_Generator/ECU_B_Error_Code_Generator/ECU_B_CAN_Error_Flags to Error_Code_Converter/Switch Case Action Subsystem1 ==
  Action Port : ActionPort  ActionPortLabel=case [ 1 ]:
  Constant : Constant  Value=800
  Out1 : Outport  VectorParamsAs1DForOutWhenUnconnected=off
  wires:
  Constant/1 -> Out1/1

== system ECU_B_Enumerated_Error_Code_Generator/ECU_B_Error_Code_Generator/ECU_B_CAN_Error_Flags to Error_Code_Converter/Switch Case Action Subsystem10 ==
  Action Port : ActionPort  ActionPortLabel=case [ 10 ]:
  Constant : Constant  Value=809
  Out1 : Outport  VectorParamsAs1DForOutWhenUnconnected=off
  wires:
  Constant/1 -> Out1/1

== system ECU_B_Enumerated_Error_Code_Generator/ECU_B_Error_Code_Generator/ECU_B_CAN_Error_Flags to Error_Code_Converter/Switch Case Action Subsystem11 ==
  Action Port : ActionPort  ActionPortLabel=case [ 11 ]:
  Constant : Constant  Value=810
  Out1 : Outport  VectorParamsAs1DForOutWhenUnconnected=off
  wires:
  Constant/1 -> Out1/1

== system ECU_B_Enumerated_Error_Code_Generator/ECU_B_Error_Code_Generator/ECU_B_CAN_Error_Flags to Error_Code_Converter/Switch Case Action Subsystem12 ==
  Action Port : ActionPort  ActionPortLabel=case [ 12 ]:
  Constant : Constant  Value=811
  Out1 : Outport  VectorParamsAs1DForOutWhenUnconnected=off
  wires:
  Constant/1 -> Out1/1

== system ECU_B_Enumerated_Error_Code_Generator/ECU_B_Error_Code_Generator/ECU_B_CAN_Error_Flags to Error_Code_Converter/Switch Case Action Subsystem13 ==
  Action Port : ActionPort  ActionPortLabel=case [ 13 ]:
  Constant : Constant  Value=812
  Out1 : Outport  VectorParamsAs1DForOutWhenUnconnected=off
  wires:
  Constant/1 -> Out1/1

== system ECU_B_Enumerated_Error_Code_Generator/ECU_B_Error_Code_Generator/ECU_B_CAN_Error_Flags to Error_Code_Converter/Switch Case Action Subsystem14 ==
  Action Port : ActionPort  ActionPortLabel=case [ 14 ]:
  Constant : Constant  Value=900
  Out1 : Outport  VectorParamsAs1DForOutWhenUnconnected=off
  wires:
  Constant/1 -> Out1/1

== system ECU_B_Enumerated_Error_Code_Generator/ECU_B_Error_Code_Generator/ECU_B_CAN_Error_Flags to Error_Code_Converter/Switch Case Action Subsystem15 ==
  Action Port : ActionPort  ActionPortLabel=case [ 17 ]:
  Constant : Constant  Value=903
  Out1 : Outport  VectorParamsAs1DForOutWhenUnconnected=off
  wires:
  Constant/1 -> Out1/1

== system ECU_B_Enumerated_Error_Code_Generator/ECU_B_Error_Code_Generator/ECU_B_CAN_Error_Flags to Error_Code_Converter/Switch Case Action Subsystem16 ==
  Action Port : ActionPort  ActionPortLabel=case [ 15 ]:
  Constant : Constant  Value=901
  Out1 : Outport  VectorParamsAs1DForOutWhenUnconnected=off
  wires:
  Constant/1 -> Out1/1

== system ECU_B_Enumerated_Error_Code_Generator/ECU_B_Error_Code_Generator/ECU_B_CAN_Error_Flags to Error_Code_Converter/Switch Case Action Subsystem17 ==
  Action Port : ActionPort  ActionPortLabel=case [ 16 ]:
  Constant : Constant  Value=902
  Out1 : Outport  VectorParamsAs1DForOutWhenUnconnected=off
  wires:
  Constant/1 -> Out1/1

== system ECU_B_Enumerated_Error_Code_Generator/ECU_B_Error_Code_Generator/ECU_B_CAN_Error_Flags to Error_Code_Converter/Switch Case Action Subsystem19 ==
  Action Port : ActionPort  ActionPortLabel=case [ 26 ]:
  Constant : Constant  Value=912
  Out1 : Outport  VectorParamsAs1DForOutWhenUnconnected=off
  wires:
  Constant/1 -> Out1/1

== system ECU_B_Enumerated_Error_Code_Generator/ECU_B_Error_Code_Generator/ECU_B_CAN_Error_Flags to Error_Code_Converter/Switch Case Action Subsystem2 ==
  Action Port : ActionPort  ActionPortLabel=case [ 2 ]:
  Constant : Constant  Value=801
  Out1 : Outport  VectorParamsAs1DForOutWhenUnconnected=off
  wires:
  Constant/1 -> Out1/1

== system ECU_B_Enumerated_Error_Code_Generator/ECU_B_Error_Code_Generator/ECU_B_CAN_Error_Flags to Error_Code_Converter/Switch Case Action Subsystem20 ==
  Action Port : ActionPort  ActionPortLabel=case [ 25 ]:
  Constant : Constant  Value=911
  Out1 : Outport  VectorParamsAs1DForOutWhenUnconnected=off
  wires:
  Constant/1 -> Out1/1

== system ECU_B_Enumerated_Error_Code_Generator/ECU_B_Error_Code_Generator/ECU_B_CAN_Error_Flags to Error_Code_Converter/Switch Case Action Subsystem21 ==
  Action Port : ActionPort  ActionPortLabel=case [ 24 ]:
  Constant : Constant  Value=910
  Out1 : Outport  VectorParamsAs1DForOutWhenUnconnected=off
  wires:
  Constant/1 -> Out1/1

== system ECU_B_Enumerated_Error_Code_Generator/ECU_B_Error_Code_Generator/ECU_B_CAN_Error_Flags to Error_Code_Converter/Switch Case Action Subsystem22 ==
  Action Port : ActionPort  ActionPortLabel=case [ 23 ]:
  Constant : Constant  Value=909
  Out1 : Outport  VectorParamsAs1DForOutWhenUnconnected=off
  wires:
  Constant/1 -> Out1/1

== system ECU_B_Enumerated_Error_Code_Generator/ECU_B_Error_Code_Generator/ECU_B_CAN_Error_Flags to Error_Code_Converter/Switch Case Action Subsystem23 ==
  Action Port : ActionPort  ActionPortLabel=case [ 22 ]:
  Constant : Constant  Value=908
  Out1 : Outport  VectorParamsAs1DForOutWhenUnconnected=off
  wires:
  Constant/1 -> Out1/1

== system ECU_B_Enumerated_Error_Code_Generator/ECU_B_Error_Code_Generator/ECU_B_CAN_Error_Flags to Error_Code_Converter/Switch Case Action Subsystem24 ==
  Action Port : ActionPort  ActionPortLabel=case [ 21 ]:
  Constant : Constant  Value=907
  Out1 : Outport  VectorParamsAs1DForOutWhenUnconnected=off
  wires:
  Constant/1 -> Out1/1

== system ECU_B_Enumerated_Error_Code_Generator/ECU_B_Error_Code_Generator/ECU_B_CAN_Error_Flags to Error_Code_Converter/Switch Case Action Subsystem25 ==
  Action Port : ActionPort  ActionPortLabel=case [ 20 ]:
  Constant : Constant  Value=906
  Out1 : Outport  VectorParamsAs1DForOutWhenUnconnected=off
  wires:
  Constant/1 -> Out1/1

== system ECU_B_Enumerated_Error_Code_Generator/ECU_B_Error_Code_Generator/ECU_B_CAN_Error_Flags to Error_Code_Converter/Switch Case Action Subsystem26 ==
  Action Port : ActionPort  ActionPortLabel=case [ 19 ]:
  Constant : Constant  Value=905
  Out1 : Outport  VectorParamsAs1DForOutWhenUnconnected=off
  wires:
  Constant/1 -> Out1/1

== system ECU_B_Enumerated_Error_Code_Generator/ECU_B_Error_Code_Generator/ECU_B_CAN_Error_Flags to Error_Code_Converter/Switch Case Action Subsystem27 ==
  Action Port : ActionPort  ActionPortLabel=case [ 18 ]:
  Constant : Constant  Value=904
  Out1 : Outport  VectorParamsAs1DForOutWhenUnconnected=off
  wires:
  Constant/1 -> Out1/1

== system ECU_B_Enumerated_Error_Code_Generator/ECU_B_Error_Code_Generator/ECU_B_CAN_Error_Flags to Error_Code_Converter/Switch Case Action Subsystem3 ==
  Action Port : ActionPort  ActionPortLabel=case [ 7 ]:
  Constant : Constant  Value=806
  Out1 : Outport  VectorParamsAs1DForOutWhenUnconnected=off
  wires:
  Constant/1 -> Out1/1

== system ECU_B_Enumerated_Error_Code_Generator/ECU_B_Error_Code_Generator/ECU_B_CAN_Error_Flags to Error_Code_Converter/Switch Case Action Subsystem4 ==
  Action Port : ActionPort  ActionPortLabel=case [ 3 ]:
  Constant : Constant  Value=802
  Out1 : Outport  VectorParamsAs1DForOutWhenUnconnected=off
  wires:
  Constant/1 -> Out1/1

== system ECU_B_Enumerated_Error_Code_Generator/ECU_B_Error_Code_Generator/ECU_B_CAN_Error_Flags to Error_Code_Converter/Switch Case Action Subsystem5 ==
  Action Port : ActionPort  ActionPortLabel=case [ 4 ]:
  Constant : Constant  Value=803
  Out1 : Outport  VectorParamsAs1DForOutWhenUnconnected=off
  wires:
  Constant/1 -> Out1/1

== system ECU_B_Enumerated_Error_Code_Generator/ECU_B_Error_Code_Generator/ECU_B_CAN_Error_Flags to Error_Code_Converter/Switch Case Action Subsystem6 ==
  Action Port : ActionPort  ActionPortLabel=case [ 5 ]:
  Constant : Constant  Value=804
  Out1 : Outport  VectorParamsAs1DForOutWhenUnconnected=off
  wires:
  Constant/1 -> Out1/1

== system ECU_B_Enumerated_Error_Code_Generator/ECU_B_Error_Code_Generator/ECU_B_CAN_Error_Flags to Error_Code_Converter/Switch Case Action Subsystem7 ==
  Action Port : ActionPort  ActionPortLabel=case [ 6 ]:
  Constant : Constant  Value=805
  Out1 : Outport  VectorParamsAs1DForOutWhenUnconnected=off
  wires:
  Constant/1 -> Out1/1

== system ECU_B_Enumerated_Error_Code_Generator/ECU_B_Error_Code_Generator/ECU_B_CAN_Error_Flags to Error_Code_Converter/Switch Case Action Subsystem8 ==
  Action Port : ActionPort  ActionPortLabel=case [ 8 ]:
  Constant : Constant  Value=807
  Out1 : Outport  VectorParamsAs1DForOutWhenUnconnected=off
  wires:
  Constant/1 -> Out1/1

== system ECU_B_Enumerated_Error_Code_Generator/ECU_B_Error_Code_Generator/ECU_B_CAN_Error_Flags to Error_Code_Converter/Switch Case Action Subsystem9 ==
  Action Port : ActionPort  ActionPortLabel=case [ 9 ]:
  Constant : Constant  Value=808
  Out1 : Outport  VectorParamsAs1DForOutWhenUnconnected=off
  wires:
  Constant/1 -> Out1/1

== system ECU_B_Enumerated_Error_Code_Generator/ECU_B_Error_Code_Generator/ECU_B_Delta_Error_Flags to Error_Code_Converter/Switch Case Action Subsystem1 ==
  Action Port : ActionPort  ActionPortLabel=case [ 1 ]:
  Constant : Constant  Value=600
  Out1 : Outport  VectorParamsAs1DForOutWhenUnconnected=off
  wires:
  Constant/1 -> Out1/1

== system ECU_B_Enumerated_Error_Code_Generator/ECU_B_Error_Code_Generator/ECU_B_Delta_Error_Flags to Error_Code_Converter/Switch Case Action Subsystem10 ==
  Action Port : ActionPort  ActionPortLabel=case [ 10 ]:
  Constant : Constant  Value=609
  Out1 : Outport  VectorParamsAs1DForOutWhenUnconnected=off
  wires:
  Constant/1 -> Out1/1

== system ECU_B_Enumerated_Error_Code_Generator/ECU_B_Error_Code_Generator/ECU_B_Delta_Error_Flags to Error_Code_Converter/Switch Case Action Subsystem11 ==
  Action Port : ActionPort  ActionPortLabel=case [ 11 ]:
  Constant : Constant  Value=610
  Out1 : Outport  VectorParamsAs1DForOutWhenUnconnected=off
  wires:
  Constant/1 -> Out1/1

== system ECU_B_Enumerated_Error_Code_Generator/ECU_B_Error_Code_Generator/ECU_B_Delta_Error_Flags to Error_Code_Converter/Switch Case Action Subsystem12 ==
  Action Port : ActionPort  ActionPortLabel=case [ 12 ]:
  Constant : Constant  Value=611
  Out1 : Outport  VectorParamsAs1DForOutWhenUnconnected=off
  wires:
  Constant/1 -> Out1/1

== system ECU_B_Enumerated_Error_Code_Generator/ECU_B_Error_Code_Generator/ECU_B_Delta_Error_Flags to Error_Code_Converter/Switch Case Action Subsystem13 ==
  Action Port : ActionPort  ActionPortLabel=case [ 13 ]:
  Constant : Constant  Value=612
  Out1 : Outport  VectorParamsAs1DForOutWhenUnconnected=off
  wires:
  Constant/1 -> Out1/1

== system ECU_B_Enumerated_Error_Code_Generator/ECU_B_Error_Code_Generator/ECU_B_Delta_Error_Flags to Error_Code_Converter/Switch Case Action Subsystem14 ==
  Action Port : ActionPort  ActionPortLabel=case [ 14 ]:
  Constant : Constant  Value=613
  Out1 : Outport  VectorParamsAs1DForOutWhenUnconnected=off
  wires:
  Constant/1 -> Out1/1

== system ECU_B_Enumerated_Error_Code_Generator/ECU_B_Error_Code_Generator/ECU_B_Delta_Error_Flags to Error_Code_Converter/Switch Case Action Subsystem15 ==
  Action Port : ActionPort  ActionPortLabel=case [ 17 ]:
  Constant : Constant  Value=700
  Out1 : Outport  VectorParamsAs1DForOutWhenUnconnected=off
  wires:
  Constant/1 -> Out1/1

== system ECU_B_Enumerated_Error_Code_Generator/ECU_B_Error_Code_Generator/ECU_B_Delta_Error_Flags to Error_Code_Converter/Switch Case Action Subsystem16 ==
  Action Port : ActionPort  ActionPortLabel=case [ 15 ]:
  Constant : Constant  Value=614
  Out1 : Outport  VectorParamsAs1DForOutWhenUnconnected=off
  wires:
  Constant/1 -> Out1/1

== system ECU_B_Enumerated_Error_Code_Generator/ECU_B_Error_Code_Generator/ECU_B_Delta_Error_Flags to Error_Code_Converter/Switch Case Action Subsystem17 ==
  Action Port : ActionPort  ActionPortLabel=case [ 16 ]:
  Constant : Constant  Value=615
  Out1 : Outport  VectorParamsAs1DForOutWhenUnconnected=off
  wires:
  Constant/1 -> Out1/1

== system ECU_B_Enumerated_Error_Code_Generator/ECU_B_Error_Code_Generator/ECU_B_Delta_Error_Flags to Error_Code_Converter/Switch Case Action Subsystem18 ==
  Action Port : ActionPort  ActionPortLabel=case [ 18 ]:
  Constant : Constant  Value=701
  Out1 : Outport  VectorParamsAs1DForOutWhenUnconnected=off
  wires:
  Constant/1 -> Out1/1

== system ECU_B_Enumerated_Error_Code_Generator/ECU_B_Error_Code_Generator/ECU_B_Delta_Error_Flags to Error_Code_Converter/Switch Case Action Subsystem19 ==
  Action Port : ActionPort  ActionPortLabel=case [ 19 ]:
  Constant : Constant  Value=702
  Out1 : Outport  VectorParamsAs1DForOutWhenUnconnected=off
  wires:
  Constant/1 -> Out1/1

== system ECU_B_Enumerated_Error_Code_Generator/ECU_B_Error_Code_Generator/ECU_B_Delta_Error_Flags to Error_Code_Converter/Switch Case Action Subsystem2 ==
  Action Port : ActionPort  ActionPortLabel=case [ 2 ]:
  Constant : Constant  Value=601
  Out1 : Outport  VectorParamsAs1DForOutWhenUnconnected=off
  wires:
  Constant/1 -> Out1/1

== system ECU_B_Enumerated_Error_Code_Generator/ECU_B_Error_Code_Generator/ECU_B_Delta_Error_Flags to Error_Code_Converter/Switch Case Action Subsystem20 ==
  Action Port : ActionPort  ActionPortLabel=case [ 21 ]:
  Constant : Constant  Value=704
  Out1 : Outport  VectorParamsAs1DForOutWhenUnconnected=off
  wires:
  Constant/1 -> Out1/1

== system ECU_B_Enumerated_Error_Code_Generator/ECU_B_Error_Code_Generator/ECU_B_Delta_Error_Flags to Error_Code_Converter/Switch Case Action Subsystem21 ==
  Action Port : ActionPort  ActionPortLabel=case [ 20 ]:
  Constant : Constant  Value=703
  Out1 : Outport  VectorParamsAs1DForOutWhenUnconnected=off
  wires:
  Constant/1 -> Out1/1

== system ECU_B_Enumerated_Error_Code_Generator/ECU_B_Error_Code_Generator/ECU_B_Delta_Error_Flags to Error_Code_Converter/Switch Case Action Subsystem22 ==
  Action Port : ActionPort  ActionPortLabel=case [ 22 ]:
  Constant : Constant  Value=705
  Out1 : Outport  VectorParamsAs1DForOutWhenUnconnected=off
  wires:
  Constant/1 -> Out1/1

== system ECU_B_Enumerated_Error_Code_Generator/ECU_B_Error_Code_Generator/ECU_B_Delta_Error_Flags to Error_Code_Converter/Switch Case Action Subsystem23 ==
  Action Port : ActionPort  ActionPortLabel=case [ 28 ]:
  Constant : Constant  Value=711
  Out1 : Outport  VectorParamsAs1DForOutWhenUnconnected=off
  wires:
  Constant/1 -> Out1/1

== system ECU_B_Enumerated_Error_Code_Generator/ECU_B_Error_Code_Generator/ECU_B_Delta_Error_Flags to Error_Code_Converter/Switch Case Action Subsystem24 ==
  Action Port : ActionPort  ActionPortLabel=case [ 32 ]:
  Constant : Constant  Value=715
  Out1 : Outport  VectorParamsAs1DForOutWhenUnconnected=off
  wires:
  Constant/1 -> Out1/1

== system ECU_B_Enumerated_Error_Code_Generator/ECU_B_Error_Code_Generator/ECU_B_Delta_Error_Flags to Error_Code_Converter/Switch Case Action Subsystem25 ==
  Action Port : ActionPort  ActionPortLabel=case [ 27 ]:
  Constant : Constant  Value=710
  Out1 : Outport  VectorParamsAs1DForOutWhenUnconnected=off
  wires:
  Constant/1 -> Out1/1

== system ECU_B_Enumerated_Error_Code_Generator/ECU_B_Error_Code_Generator/ECU_B_Delta_Error_Flags to Error_Code_Converter/Switch Case Action Subsystem26 ==
  Action Port : ActionPort  ActionPortLabel=case [ 26 ]:
  Constant : Constant  Value=709
  Out1 : Outport  VectorParamsAs1DForOutWhenUnconnected=off
  wires:
  Constant/1 -> Out1/1

== system ECU_B_Enumerated_Error_Code_Generator/ECU_B_Error_Code_Generator/ECU_B_Delta_Error_Flags to Error_Code_Converter/Switch Case Action Subsystem27 ==
  Action Port : ActionPort  ActionPortLabel=case [ 23 ]:
  Constant : Constant  Value=706
  Out1 : Outport  VectorParamsAs1DForOutWhenUnconnected=off
  wires:
  Constant/1 -> Out1/1

== system ECU_B_Enumerated_Error_Code_Generator/ECU_B_Error_Code_Generator/ECU_B_Delta_Error_Flags to Error_Code_Converter/Switch Case Action Subsystem28 ==
  Action Port : ActionPort  ActionPortLabel=case [ 25 ]:
  Constant : Constant  Value=708
  Out1 : Outport  VectorParamsAs1DForOutWhenUnconnected=off
  wires:
  Constant/1 -> Out1/1

== system ECU_B_Enumerated_Error_Code_Generator/ECU_B_Error_Code_Generator/ECU_B_Delta_Error_Flags to Error_Code_Converter/Switch Case Action Subsystem29 ==
  Action Port : ActionPort  ActionPortLabel=case [ 24 ]:
  Constant : Constant  Value=707
  Out1 : Outport  VectorParamsAs1DForOutWhenUnconnected=off
  wires:
  Constant/1 -> Out1/1

== system ECU_B_Enumerated_Error_Code_Generator/ECU_B_Error_Code_Generator/ECU_B_Delta_Error_Flags to Error_Code_Converter/Switch Case Action Subsystem3 ==
  Action Port : ActionPort  ActionPortLabel=case [ 7 ]:
  Constant : Constant  Value=606
  Out1 : Outport  VectorParamsAs1DForOutWhenUnconnected=off
  wires:
  Constant/1 -> Out1/1

== system ECU_B_Enumerated_Error_Code_Generator/ECU_B_Error_Code_Generator/ECU_B_Delta_Error_Flags to Error_Code_Converter/Switch Case Action Subsystem32 ==
  Action Port : ActionPort  ActionPortLabel=case [ 31 ]:
  Constant : Constant  Value=714
  Out1 : Outport  VectorParamsAs1DForOutWhenUnconnected=off
  wires:
  Constant/1 -> Out1/1

== system ECU_B_Enumerated_Error_Code_Generator/ECU_B_Error_Code_Generator/ECU_B_Delta_Error_Flags to Error_Code_Converter/Switch Case Action Subsystem33 ==
  Action Port : ActionPort  ActionPortLabel=case [ 30 ]:
  Constant : Constant  Value=713
  Out1 : Outport  VectorParamsAs1DForOutWhenUnconnected=off
  wires:
  Constant/1 -> Out1/1

== system ECU_B_Enumerated_Error_Code_Generator/ECU_B_Error_Code_Generator/ECU_B_Delta_Error_Flags to Error_Code_Converter/Switch Case Action Subsystem34 ==
  Action Port : ActionPort  ActionPortLabel=case [ 29 ]:
  Constant : Constant  Value=712
  Out1 : Outport  VectorParamsAs1DForOutWhenUnconnected=off
  wires:
  Constant/1 -> Out1/1

== system ECU_B_Enumerated_Error_Code_Generator/ECU_B_Error_Code_Generator/ECU_B_Delta_Error_Flags to Error_Code_Converter/Switch Case Action Subsystem4 ==
  Action Port : ActionPort  ActionPortLabel=case [ 3 ]:
  Constant : Constant  Value=602
  Out1 : Outport  VectorParamsAs1DForOutWhenUnconnected=off
  wires:
  Constant/1 -> Out1/1
